simulink model "test"  (R2024a)
settings: Solver=VariableStepAuto  StartTime=0.0  StopTime=30  RelTol=1e-3
values from neighbouring files (symbols this model uses):
  A = zeros(3,3)    [make_jacobian_abcd.m]
  B = [ -1/CBat ... (first row only)    [make_jacobian_abcd.m]
  C = [ voc_p - u0*RS_p,  -1,  -1 ]    [make_jacobian_abcd.m]
  D = -RS    [make_jacobian_abcd.m]
  iT = 0.05    [init_values.m]
  theta = [      CBat;      RS_a; RS_b; RS_c;      RTS_a; RTS_b; RTS_c;      CTS_a; CTS_b; CTS_c;      RTL_a; RTL_b; RTL_c;      CTL_a; CTL_b; CTL_c;      v0; v1; v2; v3; v4; v5  ]    [init_values.m]
  u0 = 0    [init_values.m]    (also in make_jacobian_abcd.m)
  y0 = voc - vTS0 - vTL0 - u0*RS    [make_jacobian_abcd.m]
libraries: simulink x1
settings Model: Creator=belit  LastModifiedBy=belit

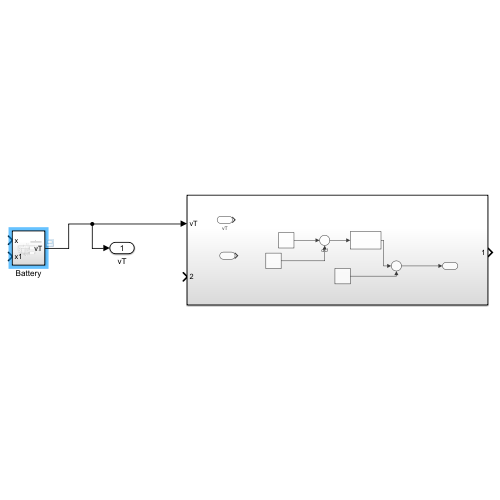
[thumbnail: Simulink's stored preview of the top-level diagram]
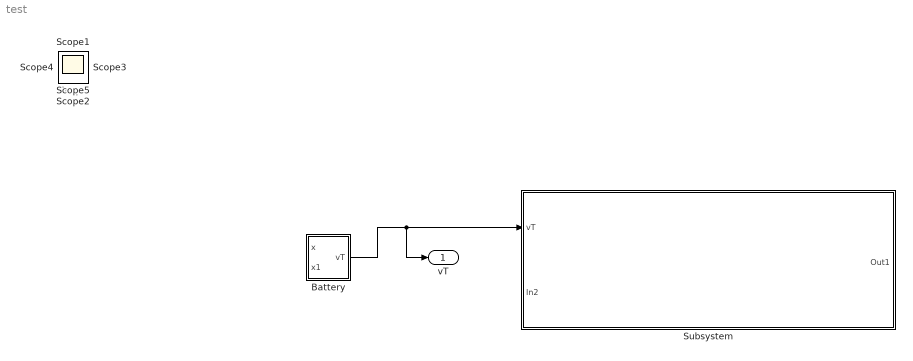
== system test ==
  Battery : Subsystem
  Subsystem : Subsystem
  vT : Outport
  Scope{,1..5} (6 alike) : Scope
  wires:
  Battery/1(vT) -> vT/1, Subsystem/1(vT)

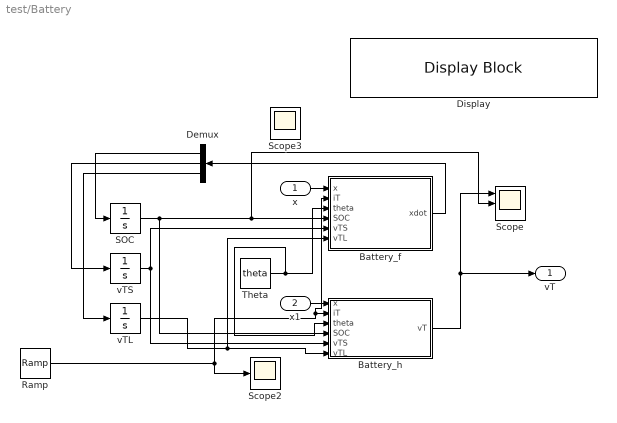
== system test/Battery ==
  x : Inport
  x1 : Inport  Port=2
  Battery_f : MATLAB Function  TreatAsAtomicUnit=on
  Battery_h : MATLAB Function  TreatAsAtomicUnit=on
  Demux : Demux  Outputs=3
  Display : DisplayBlock  Transparency=1  Layout=Fill available space
  Ramp : simulink/Sources/Ramp  slope=10  start=0  InitialOutput=0
  SOC : Integrator  InitialCondition=0.4
  Scope : Scope  NumInputPorts=3
  Scope2 : Scope
  Scope3 : Scope
  Theta : Constant  Value=theta
  vTL : Integrator  InitialCondition=0.01
  vTS : Integrator  InitialCondition=0.01
  vT : Outport
  wires:
  Battery_h/1(vT) -> vT/1, Scope/1
  Battery_f/1(xdot) -> Demux/1
  Ramp/1 -> Battery_f/2(iT), Battery_h/2(iT), Scope2/1
  SOC/1 -> Scope/2, Battery_f/4(SOC), Battery_h/4(SOC)
  vTL/1 -> Battery_h/6(vTL), Battery_f/6(vTL)
  Demux/1 -> SOC/1
  vTS/1 -> Battery_h/5(vTS), Battery_f/5(vTS)
  Theta/1 -> Battery_f/3(theta), Battery_h/3(theta)
  Demux/2 -> vTS/1
  Demux/3 -> vTL/1
  x1/1 -> Battery_h/1(x)
  x/1 -> Battery_f/1(x)

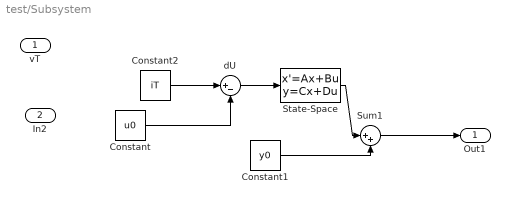
== system test/Subsystem ==
  vT : Inport
  In2 : Inport  Port=2
  Constant : Constant  Value=u0
  Constant1 : Constant  Value=y0
  Constant2 : Constant  Value=iT
  State-Space : StateSpace  A=A  B=B  C=C  D=D  InitialCondition=0
  Sum1 : Sum  Inputs=|++
  dU : Sum  Inputs=|+-
  Out1 : Outport
  wires:
  dU/1 -> State-Space/1
  Constant2/1 -> dU/1
  Constant/1 -> dU/2
  State-Space/1 -> Sum1/1
  Sum1/1 -> Out1/1
  Constant1/1 -> Sum1/2

== matlab function test/Battery/Battery_h ==
  data: x input; vT output; iT input; theta input; SOC input; vTS input; vTL input
function vT = battery_h(x, iT, theta, SOC, vTS, vTL)
%#codegen
% x = [soc; vTS; vTL], theta is 22x1 parameter vector

soc = SOC;
vTS = vTS;
vTL = vTL;

% ---- unpack theta ----
RS_a = theta(2);  RS_b = theta(3);  RS_c = theta(4);

v0 = theta(17); v1 = theta(18); v2 = theta(19);
v3 = theta(20); v4 = theta(21); v5 = theta(22);

% ---- compute ----
RS  = RS_a * exp(RS_b * soc) + RS_c;

voc = v0 * exp(v1 * soc) + v2 + v3*soc + v4*soc^2 + v5*soc^3;

vT = voc - vTS - vTL - iT * RS;
end

== matlab function test/Battery/Battery_f ==
  data: x input; xdot output; iT input; theta input; SOC input; vTS input; vTL input
function xdot = battery_f(x, iT, theta, SOC, vTS, vTL)
%#codegen
% x = [soc; vTS; vTL], theta is 22x1 parameter vector

soc = SOC;
vTS = vTS;
vTL = vTL;

% ---- unpack theta ----
CBat  = theta(1);

RS_a  = theta(2);  RS_b  = theta(3);  RS_c  = theta(4);

RTS_a = theta(5);  RTS_b = theta(6);  RTS_c = theta(7);
CTS_a = theta(8);  CTS_b = theta(9);  CTS_c = theta(10);

RTL_a = theta(11); RTL_b = theta(12); RTL_c = theta(13);
CTL_a = theta(14); CTL_b = theta(15); CTL_c = theta(16);

% ---- parameter functions ----
RTS = RTS_a * exp(RTS_b * soc) + RTS_c;
RTL = RTL_a * exp(RTL_b * soc) + RTL_c;

CTS = CTS_a * exp(CTS_b * soc) + CTS_c;
CTL = CTL_a * exp(CTL_b * soc) + CTL_c;

% guards (avoid divide-by-zero disasters)
epsC = 1e-12;
epsR = 1e-12;
if CTS < epsC, CTS = epsC; end
if CTL < epsC, CTL = epsC; end
if RTS < epsR, RTS = epsR; end
if RTL < epsR, RTL = epsR; end
if CBat < epsC, CBat = epsC; end

% ---- dynamics (slides) ----
soc_dot = -iT / CBat;
vTS_dot = -(vTS / (CTS * RTS)) + iT / CTS;
vTL_dot = -(vTL / (CTL * RTL)) + iT / CTL;

xdot = [soc_dot; vTS_dot; vTL_dot];
end
